simulink subsystem "VehicleModelRef"  (R2024a)
settings: Solver=VariableStepAuto  StartTime=0.0  StopTime=10.0  RelTol=1e-3
settings Model: Creator=drhill  LastModifiedBy=ADCL
settings SolverCC: AlgebraicLoopSolver=TrustRegion
settings OptimizationCC: ReuseModelBlockBuffer=off
settings DebuggingCC: UnconnectedInputMsg=warning  UnconnectedOutputMsg=warning  UnconnectedLineMsg=warning
settings ModelReferenceCC: EnableRefExpFcnMdlSchedulingChecks=on
settings RTWCC: GPUComputeCapability=3.5  DLArmComputeVersion=19.05

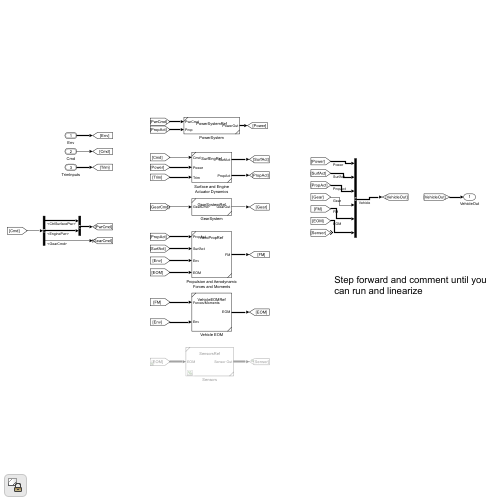
[thumbnail: Simulink's stored preview of the top-level diagram]
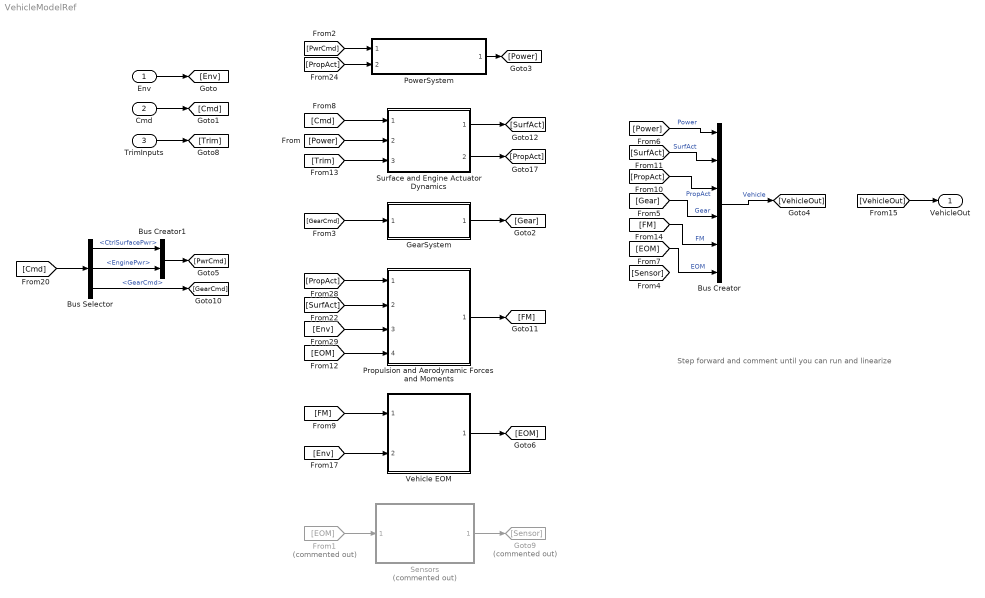
== system VehicleModelRef ==
  note: Step forward and comment until you can run and linearize
  Env : Inport  OutDataTypeStr=Bus: EnvironmentBus
  Cmd : Inport  Port=2  OutDataTypeStr=Bus: BUS_CMD
  TrimInputs : Inport  Port=3  OutDataTypeStr=Bus: BUS_TRIM_INPUT
  Bus Creator : BusCreator  Inputs=6
  Bus Creator1 : BusCreator  Inputs=2  OutDataTypeStr=Bus: BUS_POWER_SYSTEM_IN
  Bus Selector : BusSelector  OutputSignals=CtrlSurfacePwr,EnginePwr,GearCmd
  From1 : From  Commented=on  GotoTag=EOM
  GearSystem : Subsystem  ReferencedSubsystem=GearSystemRef
  Goto9 : Goto  Commented=on  GotoTag=Sensor
  PowerSystem : Subsystem  ReferencedSubsystem=PowerSystemRef
  Propulsion and Aerodynamic Forces and Moments : Subsystem  ReferencedSubsystem=AeroPropRef
  Sensors : Subsystem  Commented=on  ReferencedSubsystem=SensorsRef
  Surface and Engine Actuator Dynamics : Subsystem  ReferencedSubsystem=SurfEngRef
  Vehicle EOM : Subsystem  ReferencedSubsystem=VehicleEOMRef
  "VehicleOut " : Outport  VectorParamsAs1DForOutWhenUnconnected=off
  wires:
  Sensors/1 -> Goto9/1
  [EOM] -> Propulsion and Aerodynamic Forces and Moments/4
  [Env] -> Propulsion and Aerodynamic Forces and Moments/3
  Bus Creator/1 -> [VehicleOut]  "Vehicle"
  Propulsion and Aerodynamic Forces and Moments/1 -> [FM]
  From1/1 -> Sensors/1
  [PropAct] -> Propulsion and Aerodynamic Forces and Moments/1
  Bus Selector/1 -> Bus Creator1/1  "<CtrlSurfacePwr>"
  [PwrCmd] -> PowerSystem/1
  PowerSystem/1 -> [Power]
  [GearCmd] -> GearSystem/1
  GearSystem/1 -> [Gear]
  [Cmd] -> Surface and Engine Actuator Dynamics/1
  Bus Selector/3 -> [GearCmd]  "<GearCmd>"
  [PropAct] -> PowerSystem/2
  Cmd/1 -> [Cmd]
  [Env] -> Vehicle EOM/2
  [FM] -> Bus Creator/5  "FM"
  Env/1 -> [Env]
  [FM] -> Vehicle EOM/1
  Bus Selector/2 -> Bus Creator1/2  "<EnginePwr>"
  [Power] -> Surface and Engine Actuator Dynamics/2
  [SurfAct] -> Propulsion and Aerodynamic Forces and Moments/2
  Vehicle EOM/1 -> [EOM]
  [Cmd] -> Bus Selector/1
  TrimInputs/1 -> [Trim]
  Bus Creator1/1 -> [PwrCmd]
  [EOM] -> Bus Creator/6  "EOM"
  Surface and Engine Actuator Dynamics/1 -> [SurfAct]
  [SurfAct] -> Bus Creator/2  "SurfAct"
  [Trim] -> Surface and Engine Actuator Dynamics/3
  [Gear] -> Bus Creator/4  "Gear"
  [PropAct] -> Bus Creator/3  "PropAct"
  Surface and Engine Actuator Dynamics/2 -> [PropAct]
  [Power] -> Bus Creator/1  "Power"
  [VehicleOut] -> "VehicleOut "/1
